simulink model "Monza_simulacion_N4"  (R2018a)
settings: Solver=VariableStepAuto  StartTime=0.0  StopTime=50  FixedStep=0.033  RelTol=1e-10  AbsTol=1e-10
undefined symbols (not defined in the file or in its folder): Gain, Gain2
libraries: fuzblock x1, simulink x1
settings Model: Creator=christian  LastModifiedBy=Carlos

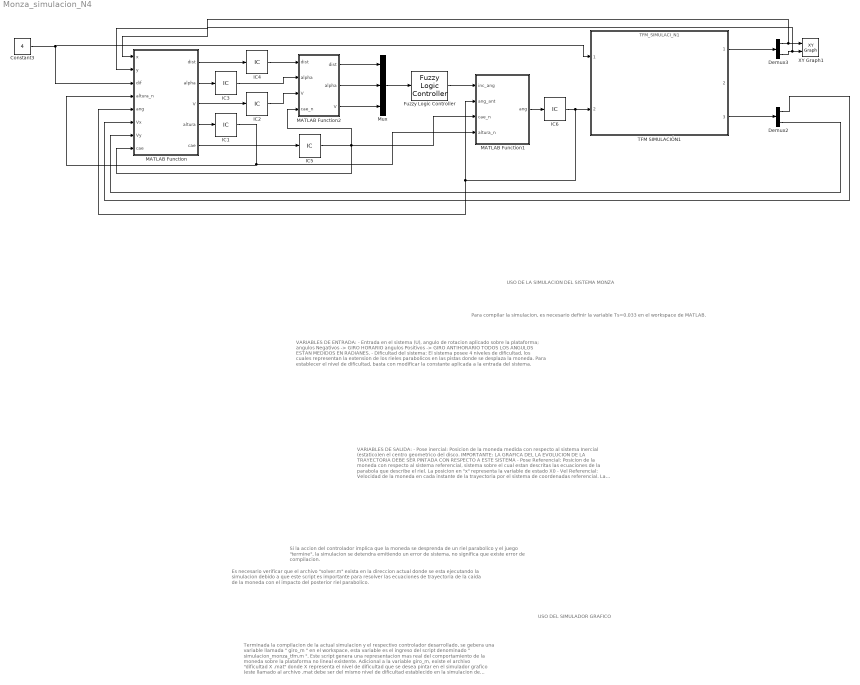
== system Monza_simulacion_N4 ==
  note: Es necesario verificar que el archivo "solver.m" exista en la direccion actual donde se esta ejecutando la simulacion debido a que este script es importante para resolver las ecuaciones de trayectoria de la caida de la moneda con el impacto del posterior riel parabolico.
  note: Si la accion del controlador implica que la moneda se desprenda de un riel parabolico y el juego "termine", la simulacion se detendra emitiendo un error de sistema, no significa que existe error de compilacion.
  note: Para compilar la simulacion, es necesario definir la variable Ts=0.033 en el workspace de MATLAB.
  note: VARIABLES DE ENTRADA:
      | - Entrada en el sistema (U), angulo de rotacion aplicado sobre la plataforma; angulos Negativos -> GIRO HORARIO
      | angulos Positivos -> GIRO ANTIHORARIO
      | TODOS LOS ANGULOS ESTAN MEDIDOS EN RADIANES.
      |
      | - Dificultad del sistema:
      | El sistema posee 4 niveles de dificultad, los cuales representan la extension de los rieles parabolicos en las pistas donde se desplaza la moneda.
      | Para establecer el nivel de dificultad, basta con modificar la constante aplicada a la entrada del sistema.
  note: USO DE LA SIMULACION DEL SISTEMA MONZA
  note: VARIABLES DE SALIDA:
      | - Pose inercial: Posicion de la moneda medida con respecto al sistema Inercial (estatico)en el centro geometrico del disco.
      | IMPORTANTE: LA GRAFICA DEL LA EVOLUCION DE LA TRAYECTORIA DEBE SER PINTADA CON RESPECTO A ESTE SISTEMA
      |
      | - Pose Referencial: Posicion de la moneda con respecto al sistema referencial, sistema sobre el cual estan descritas las ecuaciones de la parabola que describe el riel.
      | La posicion en "x" representa la variable de estado X0
      | - Vel Referencial: Velocidad de la moneda en cada instante de la trayectoria por el sistema de coordenadas referencial.
      | La velocidad en x, "x_punto" representa la variable de estado X1.
  note: USO DEL SIMULADOR GRAFICO
  note: Terminada la compilacion de la actual simulacion y el respectivo controlador desarrollado, se gebera una variable llamada " giro_m " en el workspace, esta variable es el ingreso del script denominado " simulacion_monza_tfm.m ".
      | Este script genera una representacion mas real del comportamiento de la moneda sobre la plataforma no lineal existente.
      |
      | Adicional a la variable giro_m, existe el archivo "dificultad X .mat" donde X representa el nivel de dificultad que se desea pintar en el simulador grafico (este llamado al archivo .mat debe ser del mismo nivel de dificultad establecido en la simulacion de Simulink)
  Constant3 : Constant  Value=4
  Demux2 : Demux  Outputs=2
  Demux3 : Demux  Outputs=2
  Fuzzy Logic Controller : fuzblock/Fuzzy Logic  Controller  FIS='controlador_3.fis'  OutputSampleNumber=101  DataType=double  FuzzifiedInputs=off  RuleFiringStrengths=off  RuleOutputs=off  AggregatedOutputs=off  SimulateUsing=Interpreted execution  OutOfRangeInputValueMessage=warning  NoRuleFiredMessage=warning  EmptyOutputFuzzySetMessage=warning
  IC1 : InitialCondition
  IC{2..6} (5 alike) : InitialCondition  Value=0
  MATLAB Function : MATLAB Function  TreatAsAtomicUnit=on
  MATLAB Function1 : MATLAB Function  TreatAsAtomicUnit=on
  MATLAB Function2 : MATLAB Function  TreatAsAtomicUnit=on
  Mux : Mux  Inputs=3
  TFM SIMULACIÓN1 : ModelReference  ModelNameDialog=TFM_SIMULACI_N1.slx  ParameterArgumentNames=Gain,Gain2  ParameterArgumentValues=Gain,Gain2  UsingDefaultArgumentValue=0,0  SimulationMode=Normal  ModelReferenceVersion=1.4  Gain=0  Gain2=0.0223  SimulationMode=Normal
  XY Graph1 : simulink/Sinks/XY Graph  xmin=-0.25  xmax=0.25  ymin=-0.25  ymax=0.25  st=-1
  wires:
  Demux3/1 -> MATLAB Function/1(x), XY Graph1/1
  TFM SIMULACIÓN1/1 -> Demux3/1
  Demux3/2 -> MATLAB Function/2(y), XY Graph1/2
  Constant3/1 -> TFM SIMULACIÓN1/1, MATLAB Function/3(dif)
  Demux2/1 -> MATLAB Function/6(Vx)
  TFM SIMULACIÓN1/3 -> Demux2/1
  IC1/1 -> MATLAB Function1/4(altura_n), MATLAB Function/4(altura_n)
  MATLAB Function/4(altura) -> IC1/1
  MATLAB Function/3(V) -> IC2/1
  MATLAB Function/1(dist) -> IC4/1
  MATLAB Function/2(alpha) -> IC3/1
  MATLAB Function1/1(ang) -> IC6/1
  Fuzzy Logic Controller/1 -> MATLAB Function1/1(inc_ang)
  IC6/1 -> MATLAB Function/5(ang), MATLAB Function1/2(ang_ant), TFM SIMULACIÓN1/2
  MATLAB Function/5(cae) -> IC5/1
  IC5/1 -> MATLAB Function/8("cae "), MATLAB Function2/4(cae_n), MATLAB Function1/3(cae_n)
  Mux/1 -> Fuzzy Logic Controller/1
  MATLAB Function2/1(dist) -> Mux/1
  MATLAB Function2/2(alpha) -> Mux/2
  MATLAB Function2/3(V) -> Mux/3
  IC4/1 -> MATLAB Function2/1("dist ")
  IC3/1 -> MATLAB Function2/2("alpha ")
  IC2/1 -> MATLAB Function2/3("V ")
  Demux2/2 -> MATLAB Function/7(Vy)

== matlab function Monza_simulacion_N4/MATLAB Function1 ==
  data: inc_ang input; ang output; ang_ant input; cae_n input; altura_n input
function ang = Giro_Monza(inc_ang, ang_ant, cae_n, altura_n)

movimiento = [1 0 1 0 1 0 1];
altura = round(altura_n);
cae = round(cae_n);

if movimiento(altura)==1
    inc_ang = -inc_ang;
end

umbral = 1e-3;

max = 0.2;
if cae == 0
    ang = ang_ant + inc_ang;
else
    ang = ang_ant;
end

if ang>max
    ang = max;
elseif ang<-max
    ang = -max;
elseif abs(ang)<umbral
    ang = 0;
end

== matlab function Monza_simulacion_N4/MATLAB Function ==
  data: x input; y input; dist output; dif input; alpha output; V output; altura_n input; ang input; altura output; Vx input; Vy input; cae output; cae input
function [dist,alpha,V,altura,cae] = Inclinacion(x,y,dif,altura_n,ang,Vx,Vy,cae)

umbral = 0.06;
ang = -ang;
max_Vy = 0.6;

altura = round(altura_n);


% Altura del carril
ini = 0.16;
inc = 0.0457;
alturas = zeros(1,8);
for j = 1:4
    alturas(j) = ini - (j-1)*inc;
end
for j = 5:8
    alturas(j) = -alturas(9-j);
end
alt = alturas(altura+1);

% Vectores de la posición de caida para distintas dificultades
caida = zeros(4,7,2);
caida(1,:,:) = [0 0.11429;
           0 0.06857;
           0 0.02286;
           0 -0.02286;
           0 -0.06857;
           0 -0.11429;
           -0.02554 -0.16035];
       
caida(2,:,:) = [0.06211 0.11223;
           -0.04758 0.06799;
           0.04969 0.02154;
           -0.04847 -0.02411;
           0.04406 -0.06961;
           -0.05409 -0.11585;
           -0.02554 -0.16035];
       
caida(3,:,:) = [0.12394 0.10605;
           -0.09503 0.06374;
           0.09924 0.01759;
           -0.0968 -0.02787;
           0.08803 -0.07271;
           -0.108 -0.12053;
           -0.02554 -0.16035];
       
caida(4,:,:) = [0.12394 0.10605;
           -0.14224 0.05771;
           0.14851 0.01102;
           -0.14488 -0.03412;
           0.1318 -0.07789;
           -0.108 -0.12053;
           -0.02554 -0.16035];
     

if ang~=0
    % Cambio a sistema de referencia no variable en el modo de
    % dificultad dado

    for k = 1:size(caida,2)
        x_c = caida(dif,k,1);
        y_c = caida(dif,k,2);
        distan = sqrt(x_c^2+y_c^2);
        if y_c>=0
            gamma = atan(x_c/y_c);
        elseif x_c>=0
            gamma = pi + atan(x_c/y_c);
        else
            gamma = -pi + atan(x_c/y_c);
        end

        caida(dif,k,1) = distan*sin(gamma+ang);
        caida(dif,k,2) = distan*cos(gamma+ang);
    end

    % Trigonometría
    c = cos(ang);
    s = sin(ang);
    t = tan(ang);
    t = 1/t;

    % Reducción de complejidad
    a = t - 1/(s*c);
    b = (alt + 0.463)/c;
    
    % Punto focal
    xF = (alt-0.463)*s;
    yF = (alt-0.463)*c;
    
    % Valores representativos de la parábola   
    A = 1;
    B = 2*a;
    C = a^2;
    D = -2*(xF*(a^2+1)+b*a);
    E = 2*(b-(a^2+1)*yF);
    F = (a^2+1)*xF^2 + (a^2+1)*yF^2 - b^2;
    
    valor_func = A*x^2+B*x*y+C*y^2+D*x+E*y+F;
  
    % Derivada e inclinación de un punto de recepción
    der = -(2*A*x+B*y+D)/(B*x+2*C*y+E);

else
  
    valor_func = y + 0.54*x^2 - alt;
        
    % Derivada e inclinación de un punto de recepción
    der = -2*0.54*x;

end

if ((valor_func<-umbral)&&(cae==0))%((Vy<-max_Vy)&&(cae==0))
    cae = 1;
    altura = altura+1;
elseif ((valor_func<umbral)&&(cae==1))
    cae = 0;
else
    cae = 0;
end
    
alpha = atan(der);

movimiento = [1 0 1 0 1 0 1];

% Calculo de las entradas del controlador
if movimiento(altura)==1
    dist = caida(dif,altura,1) - x;
    V = Vx;
else
    dist = x - caida(dif,altura,1);
    V = -Vx;
    alpha = -alpha;
end

== matlab function Monza_simulacion_N4/MATLAB Function2 ==
  data: dist input; alpha input; V input; dist output; cae_n input; alpha output; V output
function [dist,alpha,V] = Llamada(dist,alpha,V,cae_n)

cae = round(cae_n);

if cae==1
    dist = 0;
    alpha = -0.5;
    V = -1;
end
